simulink subsystem "JitterGen"  (R2024a)
settings: Solver=VariableStepAuto  StartTime=0.0  StopTime=10.0  RelTol=1e-3
settings Model: Creator=sjtu  LastModifiedBy=sjtu

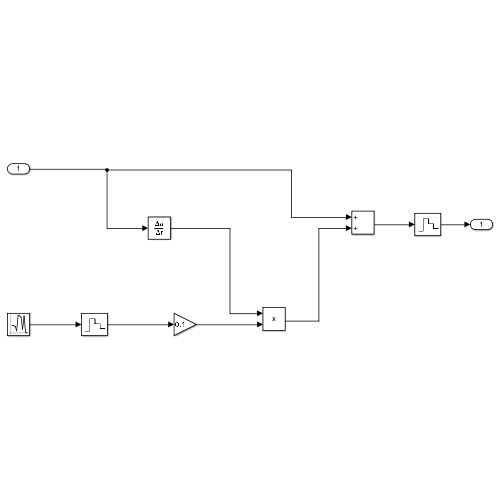
[thumbnail: Simulink's stored preview of the top-level diagram]
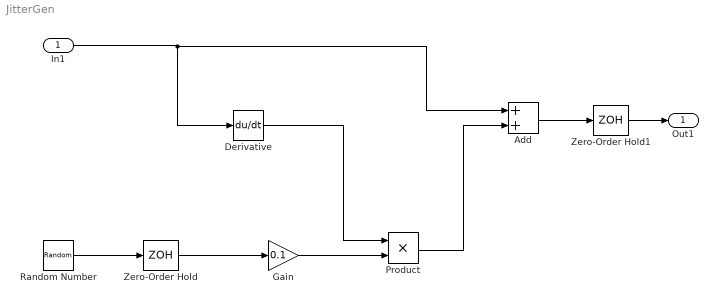
== system JitterGen ==
  In1 : Inport
  Add : Sum
  Derivative : Derivative
  Gain : Gain  Gain=0.1
  Product : Product
  Random Number : RandomNumber  SampleTime=0.1
  Zero-Order Hold : ZeroOrderHold  SampleTime=-1
  Zero-Order Hold1 : ZeroOrderHold  SampleTime=-1
  Out1 : Outport
  wires:
  Random Number/1 -> Zero-Order Hold/1
  Zero-Order Hold/1 -> Gain/1
  Gain/1 -> Product/2
  In1/1 -> Add/1, Derivative/1
  Derivative/1 -> Product/1
  Product/1 -> Add/2
  Add/1 -> Zero-Order Hold1/1
  Zero-Order Hold1/1 -> Out1/1
